simulink model "main"  (R2020b)
settings: Solver=FixedStepAuto  StartTime=0.0  StopTime=10.0  FixedStep=0.05  MaxStep=0.2  RelTol=1e-3  AbsTol=1e-3  EnableMultiTasking=on
undefined symbols (not defined in the file or in its folder): bump, steer
libraries: nesl_utility x3, sm_lib x2
settings Model: Creator=ivan  LastModifiedBy=ivan
settings SolverCC: AutoScaleAbsTol=off
settings DataIOCC: LimitDataPoints=on  MaxDataPoints=10000
settings OptimizationCC: LifeSpan=inf
settings DebuggingCC: AllowSymbolicDim=off  SFUnexpectedBacktrackingDiag=warning  SFNoUnconditionalDefaultTransitionDiag=warning  SFExecutionAtInitializationDiag=none  ArithmeticOperatorsInVariantConditions=warning
settings SFSimCC: SimUseLocalCustomCode=off  CustomCodeUndefinedFunction=UseInterfaceOnly
settings RTWCC: RTWUseLocalCustomCode=off
settings CodeAppCC: StateflowObjectComments=on
settings GRTTargetCC: TargetLangStandard=C89/C90 (ANSI)
settings ConfigComp: CovMetricSettings=dw  CovSaveCumulativeToWorkspaceVar=on  CovSaveSingleToWorkspaceVar=on  CovExternalEMLEnable=off  CovSFcnEnable=off
settings SimscapeCC: SimscapeLogType=all  SimscapeLogSimulationStatistics=on  SimscapeLogDataHistory=10000
settings ExplorerConfigSet: InternalSimMechanicsExplorerSettings="<ExplorerConfiguration><canonicalview>planar_xy</canonicalview><AnimationSetting><BasePlaybackSpeed>1.0</BasePlaybackSpeed><PlaybackSpeedFactor>1.0</PlaybackSpeedFactor></AnimationSetting><TilePanel><TileInfo><Tiles Columns=\"1\" Count=\"1\" Rows=\"1\"><Column Weight=\"1\"/><Row Weight=\"1\"/><Tile Height=\"1\" Width=\"1\" X=\"0\" Y=\"0\"/></Tiles></TileInfo><SceneInfo><SceneViewer><BGColor><R>0.60000002384185791</R><G>0.60000002384185791</G><B>0.60000002384185791</B></BGColor><Camera><DoPerspective>off</DoPerspective><Position><X>1.23625243226993642</X><Y>0.435100197498385688</Y><Z>0.40462310086390213</Z></Position><Center><X>0.414738021759955944</X><Y>0.160038738365556765</Y><Z>-0.0948318691037763617</Z></Center><Up><X>-0.041768334379467309</X><Y>0.902625507387068149</Y><Z>-0.428395377726467574</Z></Up><ViewLimDist>1</ViewLimDist><YLim>0.357454439610465358</YLim><XLim>0.359094138874733571</XLim></Camera></SceneViewer></SceneInfo></TilePanel><MechEditorPanel><Cameras/><GfxPanelCameraMap/><VideoCreator><PlaybackSpeedRatio>1.0</PlaybackSpeedRatio><FrameRate>30</FrameRate><VideoFormat>Motion JPEG AVI</VideoFormat><FrameSize>auto</FrameSize></VideoCreator></MechEditorPanel></ExplorerConfiguration>"

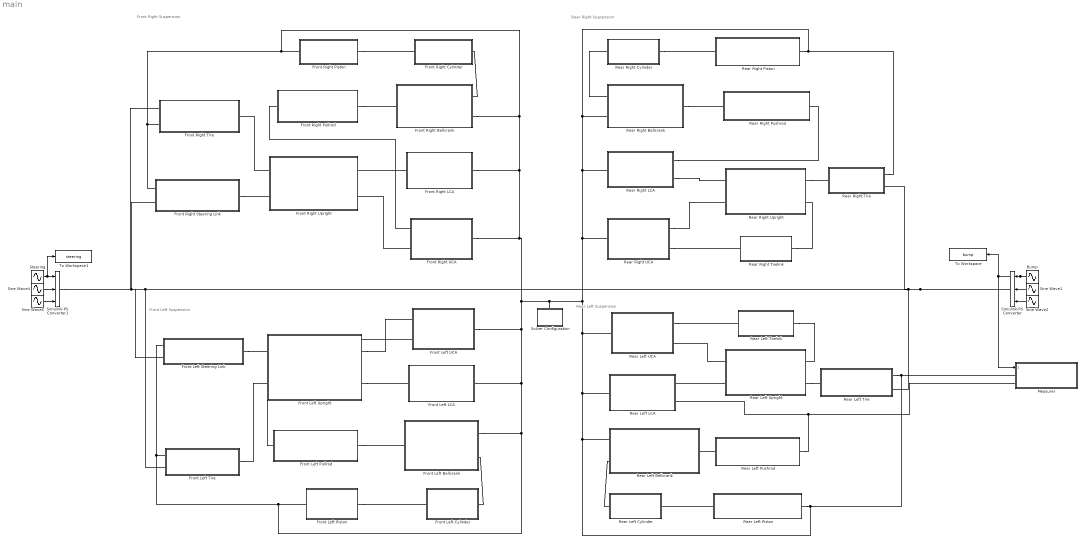
== system main ==
  note: Front Right Suspension
  note: Rear Right Suspension
  note: Front Left Suspension
  note: Rear Left Suspension
  Bump : Sin  Amplitude=bump.amp  Bias=bump.bias  Frequency=bump.freq  SampleTime=0
  Front Left Bellcrank : Subsystem  ReferencedSubsystem=Front_Left_Bellcrank
  Front Left Cylinder : Subsystem  ReferencedSubsystem=Front_Left_Cylinder
  Front Left LCA : Subsystem  ReferencedSubsystem=Front_Left_LCA
  Front Left Piston : Subsystem  ReferencedSubsystem=Front_Left_Piston
  Front Left Pullrod : Subsystem  ReferencedSubsystem=Front_Left_Pullrod
  Front Left Steering Link : Subsystem  ReferencedSubsystem=Front_Left_Steering_Link
  Front Left Tire : Subsystem  ReferencedSubsystem=Front_Left_Wheel
  Front Left UCA : Subsystem  ReferencedSubsystem=Front_Left_UCA
  Front Left Upright : Subsystem  ReferencedSubsystem=Front_Left_Upright
  Front RIght Tire : Subsystem  ReferencedSubsystem=Front_RIght_Tire
  Front Right Bellcrank : Subsystem  ReferencedSubsystem=Front_Right_Bellcrank
  Front Right Cylinder : Subsystem  ReferencedSubsystem=Front_Right_Cylinder
  Front Right LCA : Subsystem  ReferencedSubsystem=Front_Right_LCA
  Front Right Piston : Subsystem  ReferencedSubsystem=Front_Right_Piston
  Front Right Pullrod : Subsystem  ReferencedSubsystem=Front_Right_Pullrod
  Front Right Steering Link : Subsystem  ReferencedSubsystem=Front_Right_Steering_Link
  Front Right UCA : Subsystem  ReferencedSubsystem=Front_Right_UCA
  Front Right Upright : Subsystem  ReferencedSubsystem=Front_Right_Upright
  Measurer : Subsystem  ReferencedSubsystem=Measurer
  Rear Left Bellcrank : Subsystem  ReferencedSubsystem=Rear_Left_Bellcrank
  Rear Left Cylinder : Subsystem  ReferencedSubsystem=Rear_Left_Cylinder
  Rear Left LCA : Subsystem  ReferencedSubsystem=Rear_Left_LCA
  Rear Left Piston : Subsystem  ReferencedSubsystem=Rear_Left_Piston
  Rear Left Pushrod : Subsystem  ReferencedSubsystem=Rear_Left_Pushrod
  Rear Left Tire : Subsystem  ReferencedSubsystem=Rear_Left_Tire
  Rear Left Toelink : Subsystem  ReferencedSubsystem=Rear_Left_Toelink
  Rear Left UCA : Subsystem  ReferencedSubsystem=Rear_Left_UCA
  Rear Left Upright : Subsystem  ReferencedSubsystem=Rear_Left_Upright
  Rear Right Bellcrank : Subsystem  ReferencedSubsystem=Rear_Right_Bellcrank
  Rear Right Cylinder : Subsystem  ReferencedSubsystem=Rear_Right_Cylinder
  Rear Right LCA : Subsystem  ReferencedSubsystem=Rear_Right_LCA
  Rear Right Piston : Subsystem  ReferencedSubsystem=Rear_Right_Piston
  Rear Right Pushrod : Subsystem  ReferencedSubsystem=Rear_Right_Pushrod
  Rear Right Tire : Subsystem  ReferencedSubsystem=Rear_Right_Tire
  Rear Right Toelink : Subsystem  ReferencedSubsystem=Rear_Right_Toelink
  Rear Right UCA : Subsystem  ReferencedSubsystem=Rear_Right_UCA
  Rear Right Upright : Subsystem  ReferencedSubsystem=Rear_Right_Upright
  Simulink-PS Converter : nesl_utility/Simulink-PS Converter  PhysicalDomain=network_engine_domain  SubClassName=ps_input  LeftPortType=input  RightPortType=output  PseudoPeriodic=off  Frequencies=[]  NoiseDistribution=none  NoiseParameters=[]  Unit=m  AffineConversion=off  FilteringAndDerivatives=provide  SimscapeFilterOrder=1  InputFilterTimeConstant=0.001  UdotUserProvided=2
      settings: SourceProductBaseCode=PW,SS
  Simulink-PS Converter1 : nesl_utility/Simulink-PS Converter  PhysicalDomain=network_engine_domain  SubClassName=ps_input  LeftPortType=input  RightPortType=output  PseudoPeriodic=off  Frequencies=[]  NoiseDistribution=none  NoiseParameters=[]  Unit=m  AffineConversion=off  FilteringAndDerivatives=provide  SimscapeFilterOrder=1  InputFilterTimeConstant=0.001  UdotUserProvided=2
      settings: SourceProductBaseCode=PW,SS
  Sine Wave1 : Sin  Amplitude=bump.amp * bump.freq  Frequency=bump.freq  Phase=pi/2  SampleTime=0
  Sine Wave2 : Sin  Amplitude=- bump.amp * bump.freq ^ 2  Frequency=bump.freq  SampleTime=0
  Sine Wave4 : Sin  Amplitude=steer.amp * steer.freq  Frequency=steer.freq  Phase=pi/2  SampleTime=0
  Sine Wave5 : Sin  Amplitude=- steer.amp * steer.freq ^ 2  Frequency=steer.freq  SampleTime=0
  Solver Configuration : Subsystem
  Steering : Sin  Amplitude=steer.amp  Bias=steer.bias  Frequency=steer.freq  SampleTime=0
  To Workspace : ToWorkspace  VariableName=bump  SaveFormat=Timeseries  SampleTime=-1
  To Workspace1 : ToWorkspace  VariableName=steering  SaveFormat=Timeseries  SampleTime=-1
  wires:
  Sine Wave1/1 -> Simulink-PS Converter/2
  Bump/1 -> To Workspace/1, Measurer/1, Simulink-PS Converter/1
  Sine Wave2/1 -> Simulink-PS Converter/3
  Sine Wave4/1 -> Simulink-PS Converter1/2
  Steering/1 -> To Workspace1/1, Simulink-PS Converter1/1
  Sine Wave5/1 -> Simulink-PS Converter1/3
  connections:
  Front Right Steering Link/LConn1 -- Front RIght Tire/LConn2 -- Front Right Bellcrank/RConn2 -- Rear Left LCA/LConn1 -- Measurer/LConn1 -- Rear Left Tire/RConn1 -- Rear Left Piston/RConn1 -- Rear Left Bellcrank/LConn1 -- Rear Left UCA/LConn1 -- Rear Right LCA/LConn1 -- Rear Right Bellcrank/LConn2 -- Rear Right Tire/RConn1 -- Rear Right Piston/RConn1 -- Rear Right UCA/LConn1 -- Solver Configuration/LConn1 -- Front Left UCA/LConn1 -- Front Left Steering Link/LConn1 -- Front Left Tire/RConn1 -- Front Left Piston/RConn1 -- Front Left Bellcrank/LConn1 -- Front Left LCA/LConn1 -- Front Right UCA/RConn1 -- Front Right LCA/RConn1 -- Front Right Piston/RConn1
  Rear Left Toelink/RConn1 -- Rear Left Upright/RConn1
  Rear Left Upright/LConn1 -- Rear Left UCA/RConn2
  Rear Left Upright/LConn2 -- Rear Left LCA/RConn1
  Rear Left UCA/RConn1 -- Rear Left Toelink/LConn1
  Simulink-PS Converter/RConn1 -- Front RIght Tire/LConn1 -- Front Left Tire/RConn2 -- Rear Left Tire/RConn2 -- Rear Right Tire/RConn2
  Rear Left Pushrod/LConn1 -- Rear Left Bellcrank/RConn1
  Rear Left Pushrod/RConn1 -- Measurer/LConn2 -- Rear Left LCA/RConn2
  Rear Left Piston/LConn1 -- Rear Left Cylinder/RConn1
  Rear Left Cylinder/LConn1 -- Rear Left Bellcrank/LConn2
  Rear Left Upright/RConn2 -- Rear Left Tire/LConn1
  Front Left Upright/LConn1 -- Front Left UCA/RConn1
  Front Left Upright/LConn2 -- Front Left LCA/RConn1
  Front Left Steering Link/RConn1 -- Front Left Upright/RConn1
  Front Left Tire/LConn1 -- Front Left Upright/RConn2
  Simulink-PS Converter1/RConn1 -- Front Left Steering Link/LConn2 -- Front Right Steering Link/LConn2
  Front Left Pullrod/LConn1 -- Front Left Bellcrank/RConn1
  Front Left UCA/RConn2 -- Front Left Pullrod/RConn1
  Front Left Cylinder/LConn1 -- Front Left Bellcrank/LConn2
  Front Left Piston/LConn1 -- Front Left Cylinder/RConn1
  Rear Right UCA/RConn2 -- Rear Right Toelink/LConn1
  Rear Right UCA/RConn1 -- Rear Right Upright/LConn2
  Rear Right LCA/RConn2 -- Rear Right Upright/LConn1
  Rear Right LCA/RConn1 -- Rear Right Pushrod/RConn1
  Rear Right Bellcrank/RConn1 -- Rear Right Pushrod/LConn1
  Rear Right Cylinder/LConn1 -- Rear Right Bellcrank/LConn1
  Rear Right Cylinder/RConn1 -- Rear Right Piston/LConn1
  Rear Right Toelink/RConn1 -- Rear Right Upright/RConn2
  Rear Right Upright/RConn1 -- Rear Right Tire/LConn1
  Front Right UCA/LConn2 -- Front Right Upright/RConn2
  Front Right LCA/LConn1 -- Front Right Upright/RConn1
  Front Right UCA/LConn1 -- Front Right Pullrod/LConn1
  Front Right Pullrod/RConn1 -- Front Right Bellcrank/LConn1
  Front Right Steering Link/RConn1 -- Front Right Upright/LConn2
  Front Right Bellcrank/RConn1 -- Front Right Cylinder/LConn1
  Front Right Piston/LConn1 -- Front Right Cylinder/RConn1
  Front Right Upright/LConn1 -- Front RIght Tire/RConn1

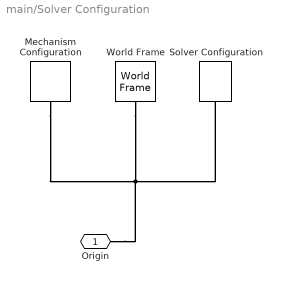
== system main/Solver Configuration ==
  Mechanism Configuration : sm_lib/Utilities/Mechanism Configuration  UniformGravity=Constant  GravityVector=[0 -9.80665 0]  GravityVectorUnits=m/s^2  GravityUnits=m/s^2  LinearizationDelta=0.001  JointModeTransitionNonlinearIterations=2
  Solver Configuration : nesl_utility/Solver Configuration  PhysicalDomain=network_engine_domain  SubClassName=solver  LeftPortType=input  RightPortType=generic  Tones=[]  Harmonics=[]  SimulateNoise=off  Profile=off  UseLocalSampling=off  EnableSwitchedLinearOptims=on  FrequencyDomain=off  UseCCode=off  RelTol=0.001  AbsTol=1e-06  MinStep=1e-09  ToWorkspace=off  RevertToSquareIcSolve=off  NumHomotopyIterations=100  PhasorMode=off  PhasorModeNumHarmonics=1  DoDC=off  ResidualTolerance=1e-09  UseLocalSolver=off  LocalSolverChoice=NE_BACKWARD_EULER_ADVANCER  LocalSolverSampleTime=0.001  DoFixedCost=off  MaxNonlinIter=3  MaxModeIter=2  ComputeImpulses=off  ImpulseIterations=2  LinearAlgebra=Sparse  EquationFormulation=NE_TIME_EF  DelaysMemoryBudget=1024  AutomaticFiltering=on  FilteringTimeConstant=0.001  PartitionStorageMethod=AS_NEEDED  PartitionMemoryBudget=1024  PartitionMethod=FAST
      settings: SourceProductName=Utilities
  World Frame : sm_lib/Frames and Transforms/World Frame
      settings: SourceProductName=Multibody
  Origin : PMIOPort  Side=Left
  connections:
  Mechanism Configuration/RConn1 -- Origin/RConn1 -- Solver Configuration/RConn1 -- World Frame/RConn1
